simulink model "zcex"  (Simulink 8.5)
settings: Solver=ode45  SolverMode=SingleTasking  StartTime=0.0  StopTime=0.1  RelTol=1e-3  AbsTol=1e-6
values from neighbouring files (symbols this model uses):
  n = abs(fix(dif/360))    [DE_12.m]
undefined symbols (not defined in the file or in its folder): b, flagc, m, minx
settings Model: Creator=PC  LastModifiedBy=PC  ExtModeTrigMode=oneshot  ExtModeArmWhenConnect=off
settings DataIOCC: LimitDataPoints=off
settings OptimizationCC: BlockReduction=off  BooleanDataType=off  ExpressionDepthLimit=128
settings DebuggingCC: SaveWithParameterizedLinksMsg=none  SignalResolutionControl=TryResolveAllWithWarning  MultiTaskDSMMsg=warning  MultiTaskCondExecSysMsg=none  FcnCallInpInsideContextMsg=EnableAllAsError  StateNameClashWarn=none  StrictBusMsg=None
settings HardwareCC: TargetUnknown=on

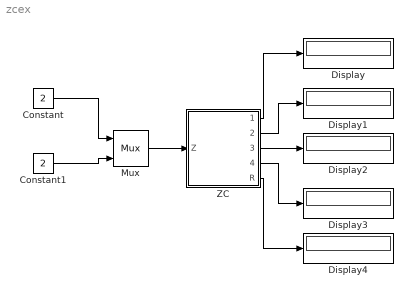
== system zcex ==
  Constant : Constant  Value=2
  Constant1 : Constant  Value=2
  Display{,1..4} (5 alike) : Display
  Mux : Mux  Inputs=2
  "ZC   " : Subsystem  mask(Zone Comparator){typez=Free expression, z1=[0 0;1 0; 1 1;0 1], z2=[0 0;2 0;2 2;0 2], z3=[0 0;3 0;3 3;0 3], z4=[0 0;4 0;4 4;0 4], zr=[0 0; -1 0; -1 -1; 0 -1], fs=4*60}
      mask prompts: typez "shape"; z1 "Zone 1"; z2 "Zone 2"; z3 "Zone 3"; z4 "Zone 4"; zr "Reverse Zone"; fs "Sampling frecuency (Hz):"
      mask help: This block performs the zone comparison. Its inputs are the resistance and reactance signals. Four forward and one backward zones are implemented. The output that corresponds to the zone where the impedance is located is set to one while the rest of the outputs are zero Either the mho or free expression characteristics may be set. For the mho characteristic, the zones are defined by specifying the center of each circle (all the circles are tangent to the origin). For the free expression, arrays with consecutive vertices specify the polygons for each zone.
      mask init:
      | zc1;
      mask Help: web(['file:///' which('zc.html')]);
      mask TypeOptions typez: Mho characteristic | Free expression
      mask Display:
      | plot(x1(:,1),x1(:,2));
      | plot(x2(:,1),x2(:,2));
      | plot(x3(:,1),x3(:,2));
      | plot(x4(:,1),x4(:,2));
      | plot(xr(:,1),xr(:,2));
  wires:
  "ZC   "/3(3) -> Display2/1
  Constant1/1 -> Mux/2
  Constant/1 -> Mux/1
  "ZC   "/1(1) -> Display/1
  "ZC   "/2(2) -> Display1/1
  "ZC   "/4(4) -> Display3/1
  "ZC   "/5(R) -> Display4/1
  Mux/1 -> "ZC   "/1(Z)

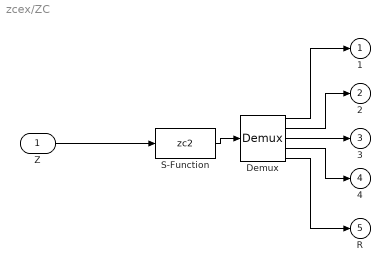
== system zcex/ZC    ==
  Z : Inport
  Demux : Demux  Outputs=5
  S-Function : S-Function  FunctionName=zc2  Parameters=z1,z2,z3,z4,zr,typez,fs,n,minx,flagc,m,b
  1 : Outport  InitialOutput=0
  2 : Outport  Port=2  InitialOutput=0
  3 : Outport  Port=3  InitialOutput=0
  4 : Outport  Port=4  InitialOutput=0
  R : Outport  Port=5  InitialOutput=0
  wires:
  Demux/5 -> R/1
  Z/1 -> S-Function/1
  Demux/4 -> 4/1
  Demux/3 -> 3/1
  Demux/2 -> 2/1
  Demux/1 -> 1/1
  S-Function/1 -> Demux/1
